simulink model "p_3_MFCm_dist"  (R2023b)
settings: Solver=ode8  StartTime=0.0  StopTime=17  FixedStep=0.001  RelTol=1e-3
values from neighbouring files (symbols this model uses):
  L1 = 0.3    [params.mat]    (also in to_be_opened_before_starting_script.mat)
  L2 = 0.2    [params.mat]    (also in to_be_opened_before_starting_script.mat)
  m1 = 4    [params.mat]    (also in to_be_opened_before_starting_script.mat)
  m2 = 3    [params.mat]    (also in to_be_opened_before_starting_script.mat)
undefined symbols (not defined in the file or in its folder): DiscIntNeverNeededParam, PARAMS, pid_MFCm_dist
libraries: slpidlib x2
settings Model: Creator=Jan Wyrwicz  LastModifiedBy=Jan Wyrwicz

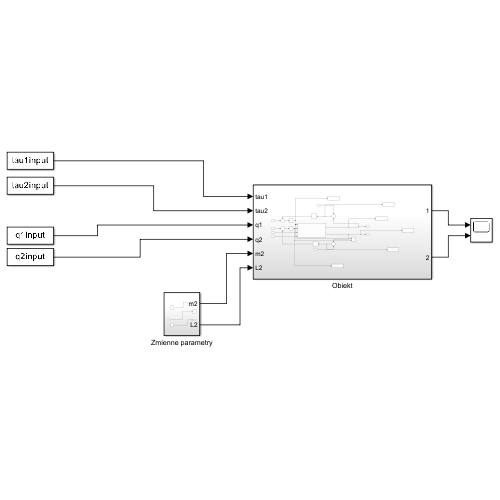
[thumbnail: Simulink's stored preview of the top-level diagram]
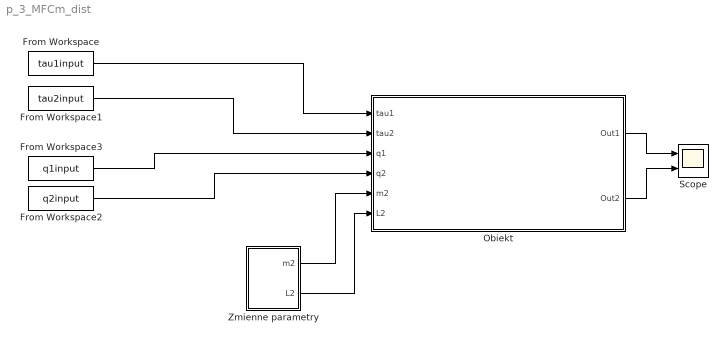
== system p_3_MFCm_dist ==
  From Workspace : FromWorkspace  VariableName=tau1input
  From Workspace1 : FromWorkspace  VariableName=tau2input
  From Workspace2 : FromWorkspace  VariableName=q2input
  From Workspace3 : FromWorkspace  VariableName=q1input
  Obiekt : Subsystem
  Scope : Scope  NumInputPorts=2
  Zmienne parametry : Subsystem
  wires:
  Obiekt/2(Out2) -> Scope/2
  Obiekt/1(Out1) -> Scope/1
  Zmienne parametry/1(m2) -> Obiekt/5(m2)
  Zmienne parametry/2(L2) -> Obiekt/6(L2)
  From Workspace2/1 -> Obiekt/4(q2)
  From Workspace3/1 -> Obiekt/3(q1)
  From Workspace1/1 -> Obiekt/2(tau2)
  From Workspace/1 -> Obiekt/1(tau1)

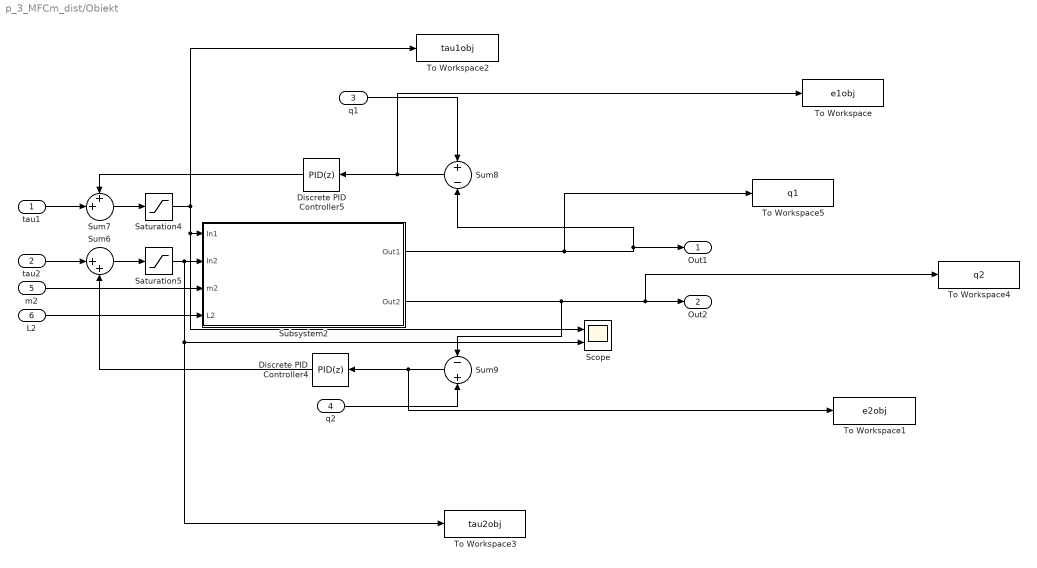
== system p_3_MFCm_dist/Obiekt ==
  tau1 : Inport
  tau2 : Inport  Port=2
  q1 : Inport  Port=3
  q2 : Inport  Port=4
  m2 : Inport  Port=5
  L2 : Inport  Port=6
  Discrete PID Controller4 : slpidlib/PID Controller  Controller=PID  Form=Parallel  TimeDomain=Discrete-time  UseExternalTs=off  SampleTime=-1  IntegratorMethod=Forward Euler  FilterMethod=Forward Euler  ControllerParametersSource=internal  P=pid_MFCm_dist(18,4)  I=pid_MFCm_dist(18,5)  UseKiTs=off  D=pid_MFCm_dist(18,6)  N=1000  UseFilter=on  TunerSelectOption=Transfer Function Based (PID Tuner App)  InitialConditionSource=internal  InitialConditionForIntegrator=0  InitialConditionForFilter=0  DifferentiatorICPrevScaledInput=0  ExternalReset=none  TrackingMode=off  Kt=1  LimitOutput=off  SatLimitsSource=internal  UpperSaturationLimit=inf  LowerSaturationLimit=-inf  LinearizeAsGain=off  AntiWindupMode=none  Kb=1  LimitIntegrator=off  UpperIntegratorSaturationLimit=inf  LowerIntegratorSaturationLimit=-inf  POutMin=[]  POutMax=[]  IOutMin=[]  IOutMax=[]  DOutMin=[]  DOutMax=[]  NOutMin=[]  NOutMax=[]  SumOutMin=[]  SumOutMax=[]  SaturationOutMin=[]  SaturationOutMax=[]  PParamMin=[]  PParamMax=[]  IParamMin=[]  IParamMax=[]  DParamMin=[]  DParamMax=[]  NParamMin=[]  NParamMax=[]  KbParamMin=[]  KbParamMax=[]  KtParamMin=[]  KtParamMax=[]  KbOutMin=[]  KbOutMax=[]  KtOutMin=[]  KtOutMax=[]  IntegratorOutMin=[]  IntegratorOutMax=[]  FilterOutMin=[]  FilterOutMax=[]  SumI1OutMin=[]  SumI1OutMax=[]  SumI2OutMin=[]  SumI2OutMax=[]  SumI3OutMin=[]  SumI3OutMax=[]  SumI4OutMin=[]  SumI4OutMax=[]  SumDOutMin=[]  SumDOutMax=[]  DifferentiatorOutMin=[]  DifferentiatorOutMax=[]  FilterDiffOutCoefMin=[]  FilterDiffOutCoefMax=[]  ReciprocalOutMin=[]  ReciprocalOutMax=[]  SumDenOutMin=[]  SumDenOutMax=[]  SumNumOutMin=[]  SumNumOutMax=[]  DivideOutMin=[]  DivideOutMax=[]  UdiffTsProdOutMin=[]  UdiffTsProdOutMax=[]  NTsProdOutMin=[]  NTsProdOutMax=[]  UintegralTsProdOutMin=[]  UintegralTsProdOutMax=[]  UngainTsProdOutMin=[]  UngainTsProdOutMax=[]  ClampingZeroOutDataTypeStr=Inherit: Inherit via back propagation  ClampingZeroOutMin=[]  ClampingZeroOutMax=[]  FilterDenConstantOutDataTypeStr=Inherit: Inherit via back propagation  FilterDenConstantOutMin=[]  FilterDenConstantOutMax=[]  PCopyOutDataTypeStr=Inherit: Inherit via back propagation  PCopyOutMin=[]  PCopyOutMax=[]  NCopyOutDataTypeStr=Inherit: Inherit via back propagation  NCopyOutMin=[]  NCopyOutMax=[]  IntegratorContinuousStateAttributes=''  IntegratorStateMustResolveToSignalObject=off  IntegratorRTWStateStorageClass=Auto  FilterContinuousStateAttributes=''  FilterStateMustResolveToSignalObject=off  FilterRTWStateStorageClass=Auto  ParallelPVariant=InternalParameters  IdealPVariant=Disabled  IVariant=InternalParameters  DVariant=InternalParameters  IntegratorVariant=Discrete  SatVariant=Disabled  AWVariant=Passthrough  PCopyVariant=Disabled  TRVariant=Disabled  FdbkBlocksVariant=Forward  IdealPFdbkVariant=Disabled  SatFdbkVariant=Disabled  DerivativeFilterVariant=ForwardEulerFilter  NVariant=InternalParameters  NCopyVariant=Disabled  FilterICVariant=InternalICsFilter  IntegratorICVariant=InternalICs  ExternalResetVariant=Disabled  TRSumVariant=Passthrough  SumFdbkVariant=Disabled  SumVariant=Sum_PID  TsampFilterVariant=InternalTs  TsampNgainVariant=Passthrough  TsampIntegralVariant=Disabled_SignalSpec  ExternalSaturationOutDataTypeStr=Inherit: Same as second input
      settings: LibrarySourceBlock=hdlsllib/Discrete/Discrete PID Controller
  Discrete PID Controller5 : slpidlib/PID Controller  Controller=PID  Form=Parallel  TimeDomain=Discrete-time  UseExternalTs=off  SampleTime=-1  IntegratorMethod=Forward Euler  FilterMethod=Forward Euler  ControllerParametersSource=internal  P=pid_MFCm_dist(18,1)  I=pid_MFCm_dist(18,2)  UseKiTs=off  D=pid_MFCm_dist(18,3)  N=1000  UseFilter=on  TunerSelectOption=Transfer Function Based (PID Tuner App)  InitialConditionSource=internal  InitialConditionForIntegrator=0  InitialConditionForFilter=0  DifferentiatorICPrevScaledInput=0  ExternalReset=none  TrackingMode=off  Kt=1  LimitOutput=off  SatLimitsSource=internal  UpperSaturationLimit=inf  LowerSaturationLimit=-inf  LinearizeAsGain=off  AntiWindupMode=none  Kb=1  LimitIntegrator=off  UpperIntegratorSaturationLimit=inf  LowerIntegratorSaturationLimit=-inf  POutMin=[]  POutMax=[]  IOutMin=[]  IOutMax=[]  DOutMin=[]  DOutMax=[]  NOutMin=[]  NOutMax=[]  SumOutMin=[]  SumOutMax=[]  SaturationOutMin=[]  SaturationOutMax=[]  PParamMin=[]  PParamMax=[]  IParamMin=[]  IParamMax=[]  DParamMin=[]  DParamMax=[]  NParamMin=[]  NParamMax=[]  KbParamMin=[]  KbParamMax=[]  KtParamMin=[]  KtParamMax=[]  KbOutMin=[]  KbOutMax=[]  KtOutMin=[]  KtOutMax=[]  IntegratorOutMin=[]  IntegratorOutMax=[]  FilterOutMin=[]  FilterOutMax=[]  SumI1OutMin=[]  SumI1OutMax=[]  SumI2OutMin=[]  SumI2OutMax=[]  SumI3OutMin=[]  SumI3OutMax=[]  SumI4OutMin=[]  SumI4OutMax=[]  SumDOutMin=[]  SumDOutMax=[]  DifferentiatorOutMin=[]  DifferentiatorOutMax=[]  FilterDiffOutCoefMin=[]  FilterDiffOutCoefMax=[]  ReciprocalOutMin=[]  ReciprocalOutMax=[]  SumDenOutMin=[]  SumDenOutMax=[]  SumNumOutMin=[]  SumNumOutMax=[]  DivideOutMin=[]  DivideOutMax=[]  UdiffTsProdOutMin=[]  UdiffTsProdOutMax=[]  NTsProdOutMin=[]  NTsProdOutMax=[]  UintegralTsProdOutMin=[]  UintegralTsProdOutMax=[]  UngainTsProdOutMin=[]  UngainTsProdOutMax=[]  ClampingZeroOutDataTypeStr=Inherit: Inherit via back propagation  ClampingZeroOutMin=[]  ClampingZeroOutMax=[]  FilterDenConstantOutDataTypeStr=Inherit: Inherit via back propagation  FilterDenConstantOutMin=[]  FilterDenConstantOutMax=[]  PCopyOutDataTypeStr=Inherit: Inherit via back propagation  PCopyOutMin=[]  PCopyOutMax=[]  NCopyOutDataTypeStr=Inherit: Inherit via back propagation  NCopyOutMin=[]  NCopyOutMax=[]  IntegratorContinuousStateAttributes=''  IntegratorStateMustResolveToSignalObject=off  IntegratorRTWStateStorageClass=Auto  FilterContinuousStateAttributes=''  FilterStateMustResolveToSignalObject=off  FilterRTWStateStorageClass=Auto  ParallelPVariant=InternalParameters  IdealPVariant=Disabled  IVariant=InternalParameters  DVariant=InternalParameters  IntegratorVariant=Discrete  SatVariant=Disabled  AWVariant=Passthrough  PCopyVariant=Disabled  TRVariant=Disabled  FdbkBlocksVariant=Forward  IdealPFdbkVariant=Disabled  SatFdbkVariant=Disabled  DerivativeFilterVariant=ForwardEulerFilter  NVariant=InternalParameters  NCopyVariant=Disabled  FilterICVariant=InternalICsFilter  IntegratorICVariant=InternalICs  ExternalResetVariant=Disabled  TRSumVariant=Passthrough  SumFdbkVariant=Disabled  SumVariant=Sum_PID  TsampFilterVariant=InternalTs  TsampNgainVariant=Passthrough  TsampIntegralVariant=Disabled_SignalSpec  ExternalSaturationOutDataTypeStr=Inherit: Same as second input
      settings: LibrarySourceBlock=hdlsllib/Discrete/Discrete PID Controller
  Saturation4 : Saturate  UpperLimit=40  LowerLimit=-40
  Saturation5 : Saturate  UpperLimit=15  LowerLimit=-15
  Scope : Scope  NumInputPorts=2
  Subsystem2 : Subsystem
  Sum6 : Sum  Inputs=|++
  Sum7 : Sum  Inputs=++|
  Sum8 : Sum  Inputs=+|-
  Sum9 : Sum  Inputs=-|+
  To Workspace : ToWorkspace  VariableName=e1obj  SampleTime=-1
      settings: Save2DSignal=2-D array (concatenate along first dimension)
  To Workspace1 : ToWorkspace  VariableName=e2obj  SampleTime=-1
      settings: Save2DSignal=2-D array (concatenate along first dimension)
  To Workspace2 : ToWorkspace  VariableName=tau1obj  SampleTime=-1
      settings: Save2DSignal=2-D array (concatenate along first dimension)
  To Workspace3 : ToWorkspace  VariableName=tau2obj  SampleTime=-1
      settings: Save2DSignal=2-D array (concatenate along first dimension)
  To Workspace4 : ToWorkspace  VariableName=q2  SampleTime=-1
      settings: Save2DSignal=2-D array (concatenate along first dimension)
  To Workspace5 : ToWorkspace  VariableName=q1  SampleTime=-1
      settings: Save2DSignal=2-D array (concatenate along first dimension)
  Out1 : Outport
  Out2 : Outport  Port=2
  wires:
  tau2/1 -> Sum6/1
  Sum6/1 -> Saturation5/1
  tau1/1 -> Sum7/2
  Sum7/1 -> Saturation4/1
  Saturation4/1 -> Scope/1, Subsystem2/1(In1), To Workspace2/1
  Saturation5/1 -> Scope/2, To Workspace3/1, Subsystem2/2(In2)
  Sum9/1 -> To Workspace1/1, Discrete PID Controller4/1
  Discrete PID Controller4/1 -> Sum6/2
  Sum8/1 -> To Workspace/1, Discrete PID Controller5/1
  Discrete PID Controller5/1 -> Sum7/1
  q1/1 -> Sum8/1
  q2/1 -> Sum9/2
  m2/1 -> Subsystem2/3(m2)
  L2/1 -> Subsystem2/4(L2)
  Subsystem2/2(Out2) -> To Workspace4/1, Out2/1, Sum9/1
  Subsystem2/1(Out1) -> To Workspace5/1, Sum8/2, Out1/1

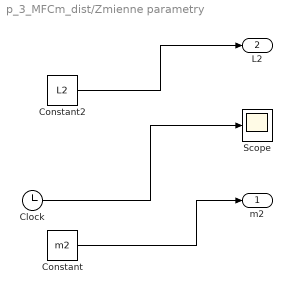
== system p_3_MFCm_dist/Zmienne parametry ==
  Clock : Clock
  Constant : Constant  Value=m2
  Constant2 : Constant  Value=L2
  Scope : Scope
  m2 : Outport
  L2 : Outport  Port=2
  wires:
  Constant/1 -> m2/1
  Clock/1 -> Scope/1
  Constant2/1 -> L2/1

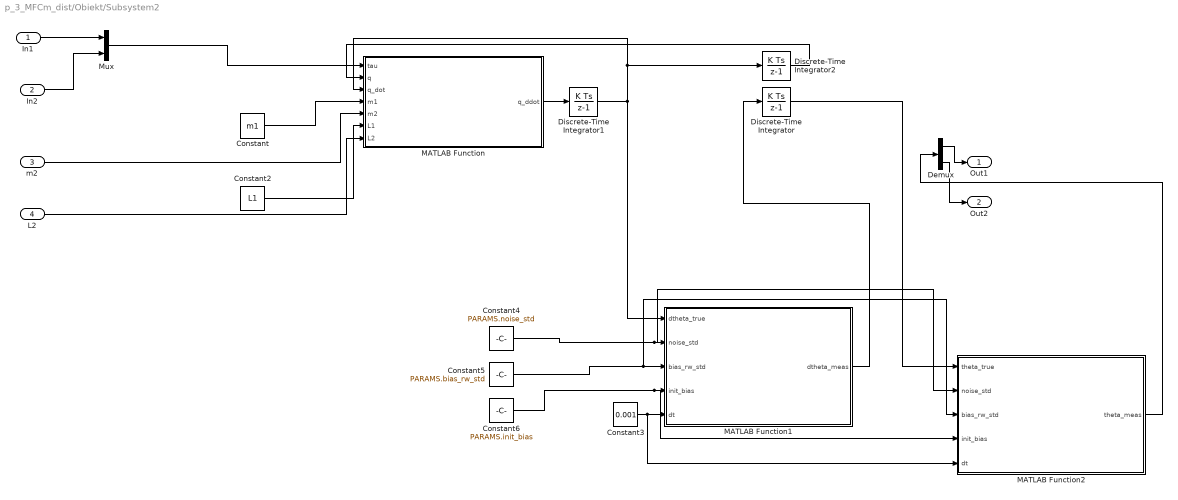
== system p_3_MFCm_dist/Obiekt/Subsystem2 ==
  In1 : Inport
  In2 : Inport  Port=2
  m2 : Inport  Port=3
  L2 : Inport  Port=4
  Constant : Constant  Value=m1
  Constant2 : Constant  Value=L1
  Constant3 : Constant  Value=0.001  SampleTime=-1
  Constant4 : Constant  Value=PARAMS.noise_std  OutDataTypeStr=double
  Constant5 : Constant  Value=PARAMS.bias_rw_std  OutDataTypeStr=double
  Constant6 : Constant  Value=PARAMS.init_bias  OutDataTypeStr=double
  Demux : Demux  Outputs=2
  Discrete-Time Integrator : DiscreteIntegrator  SampleTime=-1  ICPrevOutput=DiscIntNeverNeededParam  ICPrevScaledInput=DiscIntNeverNeededParam
  Discrete-Time Integrator1 : DiscreteIntegrator  SampleTime=-1  ICPrevOutput=DiscIntNeverNeededParam  ICPrevScaledInput=DiscIntNeverNeededParam
  Discrete-Time Integrator2 : DiscreteIntegrator  SampleTime=-1  ICPrevOutput=DiscIntNeverNeededParam  ICPrevScaledInput=DiscIntNeverNeededParam
  MATLAB Function : MATLAB Function  TreatAsAtomicUnit=on
  MATLAB Function1 : MATLAB Function  TreatAsAtomicUnit=on
  MATLAB Function2 : MATLAB Function  TreatAsAtomicUnit=on
  Mux : Mux  Inputs=2
  Out1 : Outport
  Out2 : Outport  Port=2
  wires:
  MATLAB Function/1(q_ddot) -> Discrete-Time Integrator1/1
  Mux/1 -> MATLAB Function/1(tau)
  Constant/1 -> MATLAB Function/4(m1)
  m2/1 -> MATLAB Function/5(m2)
  Constant2/1 -> MATLAB Function/6(L1)
  L2/1 -> MATLAB Function/7(L2)
  Demux/1 -> Out1/1
  Demux/2 -> Out2/1
  In1/1 -> Mux/1
  In2/1 -> Mux/2
  Discrete-Time Integrator2/1 -> MATLAB Function/2(q)
  MATLAB Function2/1(theta_meas) -> Demux/1
  Constant6/1 -> MATLAB Function2/4(init_bias), MATLAB Function1/4(init_bias)
  Discrete-Time Integrator1/1 -> MATLAB Function1/1(dtheta_true), MATLAB Function/3(q_dot), Discrete-Time Integrator2/1
  Constant3/1 -> MATLAB Function2/5(dt), MATLAB Function1/5(dt)
  Discrete-Time Integrator/1 -> MATLAB Function2/1(theta_true)
  Constant4/1 -> MATLAB Function2/2(noise_std), MATLAB Function1/2(noise_std)
  MATLAB Function1/1(dtheta_meas) -> Discrete-Time Integrator/1
  Constant5/1 -> MATLAB Function2/3(bias_rw_std), MATLAB Function1/3(bias_rw_std)

== matlab function p_3_MFCm_dist/Obiekt/Subsystem2/MATLAB Function2 ==
  data: theta_true input; theta_meas output; noise_std input; bias_rw_std input; init_bias input; dt input
function theta_meas = PositionSensor(theta_true, noise_std, bias_rw_std, init_bias, dt)
% PositionSensor  MATLAB Function block for Simulink
% Adds bias (random walk) + white Gaussian noise to a position signal.
%
% Inputs
%   theta_true : true position (scalar or vector)
%   params     : struct with fields
%                .noise_std    (measurement noise std, same units as theta)
%                .bias_rw_std  (bias random-walk std per sqrt(second))
%                .init_bias    (initial bias, scalar or vector)
%   dt         : sample time (seconds)
%
% Output
%   theta_meas : measured position = theta_true + bias + noise
%
% Notes
%   - Do not call rng inside this block. Seed RNG in model initialization script.
%   - Use fixed dt consistent with your Simulink sample time.

persistent bias sz_noise_std sz_bias_rw_std
if isempty(bias)
    bias = init_bias .* ones(size(theta_true));
    % cache stds for speed/compatibility
    sz_noise_std   = noise_std;
    sz_bias_rw_std = bias_rw_std;
end

% bias random walk: b_{k+1} = b_k + w_b,k, w_b,k ~ N(0, (bias_rw_std)^2 * dt)
bias = bias + (sz_bias_rw_std .* sqrt(dt)) .* randn(size(bias));

% measurement noise
noise = sz_noise_std .* randn(size(theta_true));

% measured position
theta_meas = theta_true + bias + noise;
end

== matlab function p_3_MFCm_dist/Obiekt/Subsystem2/MATLAB Function1 ==
  data: dtheta_true input; dtheta_meas output; noise_std input; bias_rw_std input; init_bias input; dt input
function dtheta_meas = VelocitySensor(dtheta_true, noise_std, bias_rw_std, init_bias, dt)
% PositionSensor  MATLAB Function block for Simulink
% Adds bias (random walk) + white Gaussian noise to a position signal.
%
% Inputs
%   theta_true : true position (scalar or vector)
%   params     : struct with fields
%                .noise_std    (measurement noise std, same units as theta)
%                .bias_rw_std  (bias random-walk std per sqrt(second))
%                .init_bias    (initial bias, scalar or vector)
%   dt         : sample time (seconds)
%
% Output
%   theta_meas : measured position = theta_true + bias + noise
%
% Notes
%   - Do not call rng inside this block. Seed RNG in model initialization script.
%   - Use fixed dt consistent with your Simulink sample time.

persistent bias sz_noise_std sz_bias_rw_std
if isempty(bias)
    bias = init_bias .* ones(size(dtheta_true));
    % cache stds for speed/compatibility
    sz_noise_std   = noise_std;
    sz_bias_rw_std = bias_rw_std;
end

% bias random walk: b_{k+1} = b_k + w_b,k, w_b,k ~ N(0, (bias_rw_std)^2 * dt)
bias = bias + (sz_bias_rw_std .* sqrt(dt)) .* randn(size(bias));

% measurement noise
noise = sz_noise_std .* randn(size(dtheta_true));

% measured position
dtheta_meas = dtheta_true + bias + noise;
end

== matlab function p_3_MFCm_dist/Obiekt/Subsystem2/MATLAB Function ==
  data: tau input; q_ddot output size=[2,1]; q input; q_dot input; m1 input; m2 input; L1 input; L2 input
function q_ddot  = inverse_dynamics(tau,q,q_dot,m1,m2,L1,L2)

g = 9.8067;

invM = [                          1/(L1^2*m1 + L1^2*m2 - L1^2*m2*cos(q(2))^2),                                                -(L2 + L1*cos(q(2)))/(L1^2*L2*m1 + L1^2*L2*m2 - L1^2*L2*m2*cos(q(2))^2);...
        -(L2 + L1*cos(q(2)))/(L1^2*L2*m1 + L1^2*L2*m2 - L1^2*L2*m2*cos(q(2))^2), (L1^2*m1 + L1^2*m2 + L2^2*m2 + 2*L1*L2*m2*cos(q(2)))/(- L1^2*L2^2*m2^2*cos(q(2))^2 + L1^2*L2^2*m2^2 + m1*L1^2*L2^2*m2)];


c = [-m2*L1*L2*sin(q(2))*(2*q_dot(1)*q_dot(2) + q_dot(2)^2); m2*L1*L2*q_dot(1)^2*sin(q(2))];

G = [(m1 + m2)*L1*g*cos(q(1)) + m2*g*L2*cos(q(1) + q(2));  m2*g*L2*cos(q(1) + q(2))];


q_ddot = invM*(tau - c - G);
